simulink model "AEBControlLogicUnit"  (R2025a)
settings: Solver=FixedStepAuto  StartTime=0.0  StopTime=10.0  FixedStep=0.2  RelTol=1e-3
settings Model: Creator=Rudransh  LastModifiedBy=Rudransh
settings DataIOCC: SaveOutput=off  SaveTime=off
settings OptimizationCC: DefaultParameterBehavior=Inlined  EnhancedBackFolding=on  PassReuseOutputArgsAs=Individual arguments  ZeroExternalMemoryAtStartup=off  ZeroInternalMemoryAtStartup=off  OptimizeBlockOrder=speed  DifferentSizesBufferReuse=on  OptimizationCustomize=off  EfficientTunableParamExpr=on
settings DebuggingCC: ParameterTunabilityLossMsg=error
settings SFSimCC: MATLABDynamicMemAlloc=off
settings RTWCC: SystemTargetFile=autosar.tlc  GenCodeOnly=on  PackageGeneratedCodeAndArtifacts=on  TemplateMakefile=ert_default_tmf  DataTypeReplacement=CDataTypesFixedWidth  Description=AUTOSAR
settings CodeAppCC: ForceParamTrailComments=on  IgnoreCustomStorageClasses=off  OperatorAnnotations=on  SimulinkDataObjDesc=on  SFDataObjDesc=on  InsertBlockDesc=on
settings STFCustomTargetCC: SystemTargetFile=autosar.tlc  TargetLangStandard=C99 (ISO)  MultiwordLength=256.0  DynamicStringBufferSize=256.0  ParMdlRefBuildCompliant=on  CompOptLevelCompliant=on  IncludeMdlTerminateFcn=off  CombineOutputUpdateFcns=on  SuppressErrorStatus=on  ERTCustomFileBanners=on  SupportNonFinite=off  SupportComplex=off  SupportContinuousTime=off  SupportNonInlinedSFcns=off  RemoveResetFunc=on  MATLABClassNameForMDSCustomization=Simulink.SoftwareTarget.ERTCustomization  AutosarCompliant=on  GRTInterface=off  UseToolchainInfoCompliant=on  LookupTableObjectStructAxisOrder=2,1,3,4,...  LUTObjectStructOrderEvenSpacing=Size,Table,Breakpoints  AutosarMaxShortNameLength=128.0  AutosarCompilerAbstraction=off  DisableAUTOSARRoutinesHostLibrary=off  AutosarSchemaVersion=R23-11  AutosarMatrixIOAsArray=off
settings ERTTargetCC: ExtModeTransport=0.0  ExtModeStaticAlloc=off  ExtModeMexFile=ext_comm  ExtModeIntrfLevel=Level1  ERTCustomFileTemplate=example_file_process.tlc  BooleanTrueId=TRUE  BooleanFalseId=FALSE  TargetLangStandard=C99 (ISO)  ConcurrentExecutionCompliant=off  IncludeMdlTerminateFcn=off  SuppressErrorStatus=on  SupportNonFinite=off  SupportComplex=off  ModelStepFunctionPrototypeControlCompliant=off  CPPClassGenCompliant=off  AutosarCompliant=on  LookupTableObjectStructAxisOrder=2,1,3,4,...  LUTObjectStructOrderEvenSpacing=Size,Table,Breakpoints

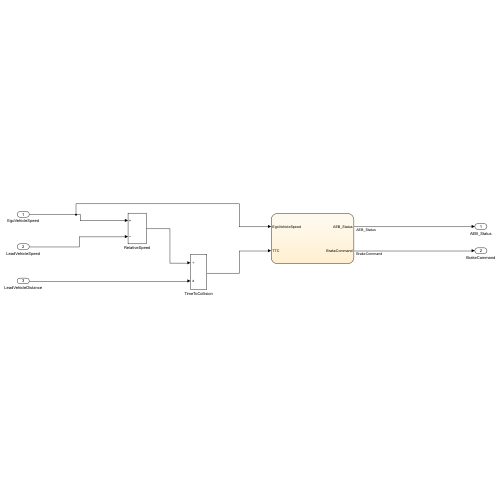
[thumbnail: Simulink's stored preview of the top-level diagram]
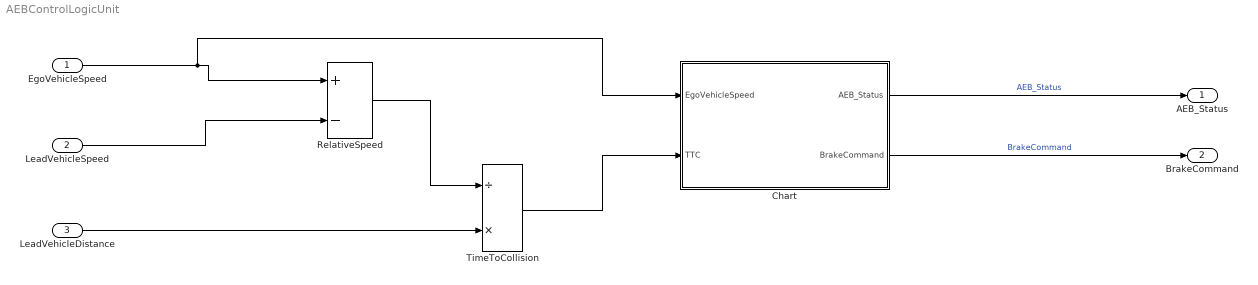
== system AEBControlLogicUnit ==
  EgoVehicleSpeed : Inport  OutDataTypeStr=double  PortDimensions=1  SampleTime=[0.20000000000000001,0]
  LeadVehicleSpeed : Inport  Port=2  OutDataTypeStr=double  PortDimensions=1  SampleTime=[0.20000000000000001,0]
  LeadVehicleDistance : Inport  Port=3  OutDataTypeStr=double  PortDimensions=1  SampleTime=[0.20000000000000001,0]
  Chart : Stateflow chart  TreatAsAtomicUnit=on
  RelativeSpeed : Sum  Inputs=+-
  TimeToCollision : Product  Inputs=/*
  AEB_Status : Outport  OutDataTypeStr=double  PortDimensions=1  SampleTime=[0.20000000000000001,0]
  BrakeCommand : Outport  Port=2  OutDataTypeStr=double  PortDimensions=1  SampleTime=[0.20000000000000001,0]
  wires:
  Chart/2(BrakeCommand) -> BrakeCommand/1  "BrakeCommand"
  Chart/1(AEB_Status) -> AEB_Status/1  "AEB_Status"
  EgoVehicleSpeed/1 -> RelativeSpeed/1, Chart/1(EgoVehicleSpeed)
  TimeToCollision/1 -> Chart/2(TTC)
  RelativeSpeed/1 -> TimeToCollision/1
  LeadVehicleSpeed/1 -> RelativeSpeed/2
  LeadVehicleDistance/1 -> TimeToCollision/2

== stateflow chart AEBControlLogicUnit/Chart ==
  state Safe
    entry: BrakeCommand = 0;
    AEB_Status = 0;
  state Warning
    entry: BrakeCommand = 0;
    AEB_Status = 1;
  state Braking
    entry: BrakeCommand = 1;
    AEB_Status = 2;
  (default) -> Safe
  Braking -> Safe : [EgoVehicleSpeed < 0.1]
  Safe -> Warning : [TTC < 2.5]
  Warning -> Safe [order 2] : [TTC >= 2.5]
  Warning -> Braking [order 1] : [TTC < 1.2]
  data: EgoVehicleSpeed input; AEB_Status output; BrakeCommand output; TTC input
